simulink model "fig85_Lampara_CFL"  (R2021a)
settings: Solver=FixedStepAuto  StartTime=0.0  StopTime=tf  FixedStep=Ts  RelTol=1e-3  EnableMultiTasking=on
InitFcn:
  | %leer señal de archivos de Excel
  | %datos = textread('Lampara_CFL.txt');
  |  datos = [
  | -1.00E-02	-2.787500E+01	1.484375E-02
  | -9.95E-03	-3.271875E+01	2.531250E-02
  | -9.90E-03	-3.375000E+01	1.015625E-02
  | -9.85E-03	-3.593750E+01	1.562500E-04
  | -9.80E-03	-4.103125E+01	1.531250E-02
  | -9.75E-03	-4.600000E+01	1.015625E-02
  | -9.70E-03	-4.828125E+01	1.562500E-04
  | -9.65E-03	-4.850000E+01	2.031250E-02
  | -9.60E-03	-5.343750E+01	1.984375E-02
  | -9.55E-03	-5.646875E+01	9.687500E-03
  | -9.50E-03	-5.756250E+01	1.046875E-02
  | -9.45E-03	-6.150000E+01	1.046875E-02
  | -9.40E-03	-6.628125E+01	9.687500E-03
  | -9.35E-03	-6.834375E+01	-1.421875E-02
  | -9.30E-03	-6.840625E+01	-3.906250E-03
  | -9.25E-03	-7.328125E+01	2.468750E-02
  | -9.20E-03	-7.637500E+01	1.500000E-02
  | -9.15E-03	-7.443750E+01	1.484375E-02
  | -9.10E-03	-7.643750E+01	3.921875E-02
  | -9.05E-03	-8.156250E+01	3.453125E-02
  | -9.00E-03	-8.156250E+01	1.953125E-02
  | -8.95E-03	-8.356250E+01	3.453125E-02
  | -8.90E-03	-8.846875E+01	2.500000E-02
  | -8.85E-03	-9.050000E+01	7.812500E-04
  | -8.80E-03	-9.550000E+01	7.812500E-04
  | -8.75E-03	-9.837500E+01	1.015625E-02
  | -8.70E-03	-1.014688E+02	-9.062500E-03
  | -8.65E-03	-1.065000E+02	-1.906250E-02
  | -8.60E-03	-1.044688E+02	-9.687500E-03
  | -8.55E-03	-1.044688E+02	-3.937500E-02
  | -8.50E-03	-1.085625E+02	-8.453125E-02
  | -8.45E-03	-1.065625E+02	-1.485938E-01
  | -8.40E-03	-1.054375E+02	-2.331250E-01
  | -8.35E-03	-1.084063E+02	-3.331250E-01
  | -8.30E-03	-1.100313E+02	-4.517188E-01
  | -8.25E-03	-1.107188E+02	-5.465625E-01
  | -8.20E-03	-1.127188E+02	-6.164063E-01
  | -8.15E-03	-1.171875E+02	-6.709375E-01
  | -8.10E-03	-1.199375E+02	-6.857813E-01
  | -8.05E-03	-1.218750E+02	-6.804688E-01
  | -8.00E-03	-1.247813E+02	-6.517188E-01
  | -7.95E-03	-1.276875E+02	-5.914063E-01
  | -7.90E-03	-1.295000E+02	-5.362500E-01
  | -7.85E-03	-1.305625E+02	-4.728125E-01
  | -7.80E-03	-1.325625E+02	-4.084375E-01
  | -7.75E-03	-1.345313E+02	-3.642188E-01
  | -7.70E-03	-1.366875E+02	-3.250000E-01
  | -7.65E-03	-1.366875E+02	-3.145313E-01
  | -7.60E-03	-1.387500E+02	-3.187500E-01
  | -7.55E-03	-1.427813E+02	-3.195313E-01
  | -7.50E-03	-1.425938E+02	-3.439063E-01
  | -7.45E-03	-1.436563E+02	-3.578125E-01
  | -7.40E-03	-1.466563E+02	-3.631250E-01
  | -7.35E-03	-1.465938E+02	-3.785938E-01
  | -7.30E-03	-1.466563E+02	-3.785938E-01
  | -7.25E-03	-1.495938E+02	-3.734375E-01
  | -7.20E-03	-1.495625E+02	-3.682813E-01
  | -7.15E-03	-1.485000E+02	-3.487500E-01
  | -7.10E-03	-1.524375E+02	-3.343750E-01
  | -7.05E-03	-1.545000E+02	-3.240625E-01
  | -7.00E-03	-1.525625E+02	-2.943750E-01
  | -6.95E-03	-1.525938E+02	-2.706250E-01
  | -6.90E-03	-1.537500E+02	-2.660938E-01
  | -6.85E-03	-1.547813E+02	-2.456250E-01
  | -6.80E-03	-1.566563E+02	-2.204688E-01
  | -6.75E-03	-1.556250E+02	-2.057813E-01
  | -6.70E-03	-1.575313E+02	-1.850000E-01
  | -6.65E-03	-1.604375E+02	-1.596875E-01
  | -6.60E-03	-1.574063E+02	-1.393750E-01
  | -6.55E-03	-1.574063E+02	-1.246875E-01
  | -6.50E-03	-1.605000E+02	-9.562500E-02
  | -6.45E-03	-1.585000E+02	-6.046875E-02
  | -6.40E-03	-1.554063E+02	-3.593750E-02
  | -6.35E-03	-1.595313E+02	-2.171875E-02
  | -6.30E-03	-1.584688E+02	-6.093750E-03
  | -6.25E-03	-1.554063E+02	4.531250E-03
  | -6.20E-03	-1.574688E+02	4.531250E-03
  | -6.15E-03	-1.564375E+02	-1.562500E-04
  | -6.10E-03	-1.553750E+02	-4.843750E-03
  | -6.05E-03	-1.554063E+02	5.000000E-03
  | -6.00E-03	-1.564375E+02	1.437500E-02
  | -5.95E-03	-1.554063E+02	1.906250E-02
  | -5.90E-03	-1.533438E+02	3.921875E-02
  | -5.85E-03	-1.543438E+02	3.875000E-02
  | -5.80E-03	-1.553750E+02	3.375000E-02
  | -5.75E-03	-1.543438E+02	4.390625E-02
  | -5.70E-03	-1.533438E+02	2.875000E-02
  | -5.65E-03	-1.524063E+02	2.421875E-02
  | -5.60E-03	-1.505000E+02	2.953125E-02
  | -5.55E-03	-1.486563E+02	1.953125E-02
  | -5.50E-03	-1.466875E+02	1.484375E-02
  | -5.45E-03	-1.447813E+02	1.484375E-02
  | -5.40E-03	-1.458125E+02	5.468750E-03
  | -5.35E-03	-1.447500E+02	5.468750E-03
  | -5.30E-03	-1.428750E+02	9.687500E-03
  | -5.25E-03	-1.447813E+02	3.125000E-04
  | -5.20E-03	-1.426250E+02	1.062500E-02
  | -5.15E-03	-1.396875E+02	1.484375E-02
  | -5.10E-03	-1.385938E+02	1.484375E-02
  | -5.05E-03	-1.375313E+02	2.000000E-02
  | -5.00E-03	-1.355625E+02	9.687500E-03
  | -4.95E-03	-1.335625E+02	4.843750E-03
  | -4.90E-03	-1.344688E+02	1.500000E-02
  | -4.85E-03	-1.337188E+02	1.468750E-02
  | -4.80E-03	-1.329688E+02	-3.125000E-04
  | -4.75E-03	-1.357188E+02	9.843750E-03
  | -4.70E-03	-1.328438E+02	1.984375E-02
  | -4.65E-03	-1.301250E+02	9.687500E-03
  | -4.60E-03	-1.330000E+02	-3.125000E-04
  | -4.55E-03	-1.289375E+02	1.500000E-02
  | -4.50E-03	-1.250313E+02	1.984375E-02
  | -4.45E-03	-1.260625E+02	-5.468750E-03
  | -4.40E-03	-1.242188E+02	4.687500E-03
  | -4.35E-03	-1.223438E+02	1.953125E-02
  | -4.30E-03	-1.206563E+02	4.218750E-03
  | -4.25E-03	-1.190625E+02	4.218750E-03
  | -4.20E-03	-1.171875E+02	1.437500E-02
  | -4.15E-03	-1.155000E+02	4.218750E-03
  | -4.10E-03	-1.137500E+02	4.218750E-03
  | -4.05E-03	-1.086875E+02	9.375000E-03
  | -4.00E-03	-1.086875E+02	4.218750E-03
  | -3.95E-03	-1.077188E+02	-9.375000E-04
  | -3.90E-03	-1.037188E+02	4.218750E-03
  | -3.85E-03	-1.017500E+02	1.437500E-02
  | -3.80E-03	-9.671875E+01	4.218750E-03
  | -3.75E-03	-9.468750E+01	-9.375000E-04
  | -3.70E-03	-9.162500E+01	-9.375000E-04
  | -3.65E-03	-8.553125E+01	4.218750E-03
  | -3.60E-03	-8.350000E+01	-9.375000E-04
  | -3.55E-03	-8.143750E+01	-6.093750E-03
  | -3.50E-03	-7.840625E+01	1.875000E-02
  | -3.45E-03	-7.546875E+01	2.328125E-02
  | -3.40E-03	-7.353125E+01	1.375000E-02
  | -3.35E-03	-7.159375E+01	1.890625E-02
  | -3.30E-03	-6.759375E+01	1.828125E-02
  | -3.25E-03	-6.665625E+01	8.750000E-03
  | -3.20E-03	-6.378125E+01	9.375000E-03
  | -3.15E-03	-5.981250E+01	4.218750E-03
  | -3.10E-03	-5.981250E+01	-7.812500E-04
  | -3.05E-03	-5.371875E+01	1.437500E-02
  | -3.00E-03	-4.659375E+01	1.437500E-02
  | -2.95E-03	-4.753125E+01	4.531250E-03
  | -2.90E-03	-4.531250E+01	1.437500E-02
  | -2.85E-03	-3.809375E+01	9.375000E-03
  | -2.80E-03	-3.700000E+01	-4.687500E-04
  | -2.75E-03	-3.706250E+01	4.375000E-03
  | -2.70E-03	-3.221875E+01	-4.687500E-04
  | -2.65E-03	-2.925000E+01	-4.687500E-04
  | -2.60E-03	-2.931250E+01	-4.687500E-04
  | -2.55E-03	-2.746875E+01	4.375000E-03
  | -2.50E-03	-2.259375E+01	1.437500E-02
  | -2.45E-03	-2.153125E+01	1.437500E-02
  | -2.40E-03	-2.240625E+01	1.437500E-02
  | -2.35E-03	-1.550000E+01	1.937500E-02
  | -2.30E-03	-9.437500E+00	2.890625E-02
  | -2.25E-03	-7.437500E+00	1.390625E-02
  | -2.20E-03	-2.531250E+00	-4.687500E-04
  | -2.15E-03	1.437500E+00	9.062500E-03
  | -2.10E-03	5.156250E+00	4.062500E-03
  | -2.05E-03	7.875000E+00	-9.375000E-04
  | -2.00E-03	9.000000E+00	-5.781250E-03
  | -1.95E-03	1.181250E+01	-9.375000E-04
  | -1.90E-03	1.356250E+01	1.812500E-02
  | -1.85E-03	1.375000E+01	4.062500E-03
  | -1.80E-03	1.484375E+01	-5.000000E-03
  | -1.75E-03	1.678125E+01	4.531250E-03
  | -1.70E-03	1.878125E+01	-4.687500E-03
  | -1.65E-03	2.168750E+01	-1.421875E-02
  | -1.60E-03	2.456250E+01	-5.000000E-03
  | -1.55E-03	2.959375E+01	9.375000E-03
  | -1.50E-03	3.446875E+01	4.531250E-03
  | -1.45E-03	3.731250E+01	4.062500E-03
  | -1.40E-03	4.143750E+01	2.812500E-02
  | -1.35E-03	4.440625E+01	2.812500E-02
  | -1.30E-03	4.728125E+01	1.859375E-02
  | -1.25E-03	4.940625E+01	2.359375E-02
  | -1.20E-03	5.040625E+01	1.859375E-02
  | -1.15E-03	5.231250E+01	2.312500E-02
  | -1.10E-03	5.631250E+01	1.859375E-02
  | -1.05E-03	5.818750E+01	9.062500E-03
  | -1.00E-03	5.912500E+01	1.812500E-02
  | -9.50E-04	6.403125E+01	1.359375E-02
  | -9.00E-04	6.900000E+01	1.859375E-02
  | -8.50E-04	7.303125E+01	2.765625E-02
  | -8.00E-04	7.403125E+01	1.812500E-02
  | -7.50E-04	7.621875E+01	2.312500E-02
  | -7.00E-04	8.128125E+01	2.765625E-02
  | -6.50E-04	8.240625E+01	1.359375E-02
  | -6.00E-04	8.146875E+01	9.062500E-03
  | -5.50E-04	8.340625E+01	1.359375E-02
  | -5.00E-04	8.653125E+01	-1.562500E-04
  | -4.50E-04	8.746875E+01	3.125000E-04
  | -4.00E-04	9.037500E+01	4.843750E-03
  | -3.50E-04	9.334375E+01	-4.687500E-03
  | -3.00E-04	9.318750E+01	4.843750E-03
  | -2.50E-04	9.712500E+01	1.515625E-02
  | -2.00E-04	9.909375E+01	5.015625E-02
  | -1.50E-04	9.606250E+01	1.189063E-01
  | -1.00E-04	9.809375E+01	1.842188E-01
  | -5.00E-05	1.011875E+02	2.790625E-01
  | 0.00E+00	9.915625E+01	4.071875E-01
  | 5.00E-05	1.001563E+02	5.062500E-01
  | 1.00E-04	1.062813E+02	5.756250E-01
  | 1.50E-04	1.074688E+02	6.493750E-01
  | 2.00E-04	1.077500E+02	6.881250E-01
  | 2.50E-04	1.136563E+02	6.929688E-01
  | 3.00E-04	1.177500E+02	6.739063E-01
  | 3.50E-04	1.199063E+02	6.246875E-01
  | 4.00E-04	1.236563E+02	5.898438E-01
  | 4.50E-04	1.267500E+02	5.160938E-01
  | 5.00E-04	1.286250E+02	4.479688E-01
  | 5.50E-04	1.296875E+02	3.882813E-01
  | 6.00E-04	1.300938E+02	3.834375E-01
  | 6.50E-04	1.300938E+02	3.590625E-01
  | 7.00E-04	1.304688E+02	3.440625E-01
  | 7.50E-04	1.304688E+02	3.489063E-01
  | 8.00E-04	1.323750E+02	3.342188E-01
  | 8.50E-04	1.346563E+02	3.587500E-01
  | 9.00E-04	1.354688E+02	3.637500E-01
  | 9.50E-04	1.374375E+02	3.840625E-01
  | 1.00E-03	1.397188E+02	3.890625E-01
  | 1.05E-03	1.407813E+02	3.840625E-01
  | 1.10E-03	1.408750E+02	3.742188E-01
  | 1.15E-03	1.448750E+02	3.581250E-01
  | 1.20E-03	1.488125E+02	3.479688E-01
  | 1.25E-03	1.478750E+02	3.431250E-01
  | 1.30E-03	1.498438E+02	3.065625E-01
  | 1.35E-03	1.535938E+02	2.915625E-01
  | 1.40E-03	1.535938E+02	2.868750E-01
  | 1.45E-03	1.509063E+02	2.617188E-01
  | 1.50E-03	1.518125E+02	2.470313E-01
  | 1.55E-03	1.545625E+02	2.281250E-01
  | 1.60E-03	1.517500E+02	2.143750E-01
  | 1.65E-03	1.507188E+02	2.092188E-01
  | 1.70E-03	1.516250E+02	1.845313E-01
  | 1.75E-03	1.496875E+02	1.553125E-01
  | 1.80E-03	1.486563E+02	1.304688E-01
  | 1.85E-03	1.496875E+02	1.053125E-01
  | 1.90E-03	1.496875E+02	7.484375E-02
  | 1.95E-03	1.496563E+02	3.984375E-02
  | 2.00E-03	1.517188E+02	2.000000E-02
  | 2.05E-03	1.536563E+02	1.500000E-02
  | 2.10E-03	1.566875E+02	9.843750E-03
  | 2.15E-03	1.568750E+02	-1.078125E-02
  | 2.20E-03	1.547813E+02	-1.578125E-02
  | 2.25E-03	1.556875E+02	-4.687500E-04
  | 2.30E-03	1.557813E+02	-5.781250E-03
  | 2.35E-03	1.517188E+02	-2.140625E-02
  | 2.40E-03	1.477813E+02	-2.140625E-02
  | 2.45E-03	1.486875E+02	-5.781250E-03
  | 2.50E-03	1.467188E+02	-1.109375E-02
  | 2.55E-03	1.448438E+02	-2.671875E-02
  | 2.60E-03	1.446563E+02	-1.640625E-02
  | 2.65E-03	1.416250E+02	-1.640625E-02
  | 2.70E-03	1.426250E+02	-1.640625E-02
  | 2.75E-03	1.406875E+02	-1.140625E-02
  | 2.80E-03	1.407188E+02	-1.140625E-02
  | 2.85E-03	1.428438E+02	-7.812500E-04
  | 2.90E-03	1.411250E+02	-1.109375E-02
  | 2.95E-03	1.440000E+02	-1.640625E-02
  | 3.00E-03	1.420313E+02	-6.093750E-03
  | 3.05E-03	1.392188E+02	-1.109375E-02
  | 3.10E-03	1.410000E+02	-1.109375E-02
  | 3.15E-03	1.369375E+02	-1.140625E-02
  | 3.20E-03	1.340938E+02	-7.812500E-04
  | 3.25E-03	1.360313E+02	9.843750E-03
  | 3.30E-03	1.358750E+02	4.531250E-03
  | 3.35E-03	1.330313E+02	-3.125000E-04
  | 3.40E-03	1.331875E+02	-5.781250E-03
  | 3.45E-03	1.329688E+02	1.000000E-02
  | 3.50E-03	1.299375E+02	5.000000E-03
  | 3.55E-03	1.290313E+02	4.218750E-03
  | 3.60E-03	1.299375E+02	2.531250E-02
  | 3.65E-03	1.288438E+02	2.546875E-02
  | 3.70E-03	1.256563E+02	3.000000E-02
  | 3.75E-03	1.253750E+02	3.062500E-02
  | 3.80E-03	1.253750E+02	2.546875E-02
  | 3.85E-03	1.232813E+02	2.015625E-02
  | 3.90E-03	1.199375E+02	2.078125E-02
  | 3.95E-03	1.177500E+02	2.078125E-02
  | 4.00E-03	1.158125E+02	2.078125E-02
  | 4.05E-03	1.138125E+02	2.078125E-02
  | 4.10E-03	1.105625E+02	2.078125E-02
  | 4.15E-03	1.045625E+02	1.531250E-02
  | 4.20E-03	1.046875E+02	4.375000E-03
  | 4.25E-03	1.036250E+02	1.468750E-02
  | 4.30E-03	9.862500E+01	-1.406250E-03
  | 4.35E-03	9.762500E+01	-1.171875E-02
  | 4.40E-03	9.559375E+01	9.218750E-03
  | 4.45E-03	9.465625E+01	-1.406250E-03
  | 4.50E-03	9.156250E+01	-9.375000E-04
  | 4.55E-03	8.643750E+01	9.843750E-03
  | 4.60E-03	8.656250E+01	1.937500E-02
  | 4.65E-03	8.462500E+01	2.484375E-02
  | 4.70E-03	7.862500E+01	4.375000E-03
  | 4.75E-03	7.568750E+01	-1.718750E-03
  | 4.80E-03	7.375000E+01	-1.718750E-03
  | 4.85E-03	7.084375E+01	-6.406250E-03
  | 4.90E-03	6.887500E+01	-1.187500E-02
  | 4.95E-03	6.596875E+01	-1.187500E-02
  | 5.00E-03	6.409375E+01	-9.375000E-04
  | 5.05E-03	6.315625E+01	1.406250E-02
  | 5.10E-03	5.906250E+01	8.593750E-03
  | 5.15E-03	5.593750E+01	-9.375000E-04
  | 5.20E-03	5.493750E+01	9.218750E-03
  | 5.25E-03	5.175000E+01	-1.562500E-03
  | 5.30E-03	4.956250E+01	3.437500E-03
  | 5.35E-03	4.671875E+01	1.437500E-02
  | 5.40E-03	4.481250E+01	3.750000E-03
  | 5.45E-03	4.284375E+01	1.859375E-02
  | 5.50E-03	3.806250E+01	2.390625E-02
  | 5.55E-03	3.525000E+01	9.218750E-03
  | 5.60E-03	3.231250E+01	9.218750E-03
  | 5.65E-03	2.828125E+01	1.406250E-02
  | 5.70E-03	2.434375E+01	4.531250E-03
  | 5.75E-03	2.137500E+01	-5.156250E-03
  | 5.80E-03	1.831250E+01	-3.125000E-04
  | 5.85E-03	1.534375E+01	9.531250E-03
  | 5.90E-03	1.334375E+01	-1.562500E-04
  | 5.95E-03	1.034375E+01	-1.000000E-02
  | 6.00E-03	6.437500E+00	9.843750E-03
  | 6.05E-03	3.593750E+00	9.843750E-03
  | 6.10E-03	7.187500E-01	0.000000E+00
  | 6.15E-03	-2.218750E+00	5.000000E-03
  | 6.20E-03	-5.250000E+00	4.687500E-03
  | 6.25E-03	-7.250000E+00	9.531250E-03
  | 6.30E-03	-9.062500E+00	4.687500E-03
  | 6.35E-03	-1.296875E+01	4.687500E-03
  | 6.40E-03	-1.600000E+01	9.531250E-03
  | 6.45E-03	-1.781250E+01	9.531250E-03
  | 6.50E-03	-2.368750E+01	9.843750E-03
  | 6.55E-03	-2.753125E+01	-3.125000E-04
  | 6.60E-03	-2.753125E+01	-6.250000E-04
  | 6.65E-03	-3.359375E+01	-5.468750E-03
  | 6.70E-03	-3.743750E+01	-2.046875E-02
  | 6.75E-03	-3.553125E+01	-1.046875E-02
  | 6.80E-03	-3.853125E+01	4.531250E-03
  | 6.85E-03	-4.540625E+01	-1.046875E-02
  | 6.90E-03	-4.643750E+01	-1.531250E-02
  | 6.95E-03	-4.546875E+01	4.687500E-03
  | 7.00E-03	-5.134375E+01	-6.250000E-04
  | 7.05E-03	-5.712500E+01	-1.046875E-02
  | 7.10E-03	-5.721875E+01	-3.125000E-04
  | 7.15E-03	-5.918750E+01	-6.250000E-04
  | 7.20E-03	-6.300000E+01	-5.468750E-03
  | 7.25E-03	-6.600000E+01	4.687500E-03
  | 7.30E-03	-6.800000E+01	4.531250E-03
  | 7.35E-03	-7.015625E+01	-1.046875E-02
  | 7.40E-03	-7.537500E+01	-3.125000E-04
  | 7.45E-03	-7.515625E+01	-6.250000E-04
  | 7.50E-03	-7.421875E+01	-1.078125E-02
  | 7.55E-03	-8.165625E+01	-5.625000E-03
  | 7.60E-03	-8.450000E+01	-5.625000E-03
  | 7.65E-03	-8.240625E+01	-6.250000E-04
  | 7.70E-03	-8.659375E+01	4.531250E-03
  | 7.75E-03	-9.156250E+01	-6.250000E-04
  | 7.80E-03	-9.362500E+01	-6.250000E-04
  | 7.85E-03	-9.565625E+01	4.531250E-03
  | 7.90E-03	-9.756250E+01	-6.250000E-04
  | 7.95E-03	-9.959375E+01	-5.625000E-03
  | 8.00E-03	-1.006563E+02	-5.625000E-03
  | 8.05E-03	-1.025313E+02	-5.625000E-03
  | 8.10E-03	-1.044375E+02	-2.125000E-02
  | 8.15E-03	-1.035000E+02	-6.125000E-02
  | 8.20E-03	-1.043750E+02	-1.154688E-01
  | 8.25E-03	-1.072500E+02	-1.965625E-01
  | 8.30E-03	-1.083125E+02	-3.007813E-01
  | 8.35E-03	-1.082813E+02	-4.087500E-01
  | 8.40E-03	-1.104375E+02	-5.192188E-01
  | 8.45E-03	-1.136250E+02	-5.989063E-01
  | 8.50E-03	-1.136563E+02	-6.526563E-01
  | 8.55E-03	-1.167188E+02	-6.971875E-01
  | 8.60E-03	-1.189063E+02	-6.973438E-01
  | 8.65E-03	-1.199688E+02	-6.631250E-01
  | 8.70E-03	-1.246875E+02	-6.184375E-01
  | 8.75E-03	-1.276563E+02	-5.640625E-01
  | 8.80E-03	-1.316875E+02	-4.990625E-01
  | 8.85E-03	-1.325938E+02	-4.392188E-01
  | 8.90E-03	-1.345938E+02	-3.953125E-01
  | 8.95E-03	-1.395313E+02	-3.546875E-01
  | 9.00E-03	-1.385313E+02	-3.289063E-01
  | 9.05E-03	-1.375313E+02	-3.242188E-01
  | 9.10E-03	-1.415313E+02	-3.192188E-01
  | 9.15E-03	-1.435625E+02	-3.343750E-01
  | 9.20E-03	-1.405938E+02	-3.492188E-01
  | 9.25E-03	-1.425938E+02	-3.548438E-01
  | 9.30E-03	-1.466250E+02	-3.862500E-01
  | 9.35E-03	-1.445938E+02	-3.959375E-01
  | 9.40E-03	-1.453438E+02	-4.014063E-01
  | 9.45E-03	-1.483438E+02	-3.967188E-01
  | 9.50E-03	-1.492813E+02	-3.607813E-01
  | 9.55E-03	-1.508125E+02	-3.414063E-01
  | 9.60E-03	-1.516250E+02	-3.256250E-01
  | 9.65E-03	-1.508438E+02	-2.895313E-01
  | 9.70E-03	-1.516250E+02	-2.507813E-01
  | 9.75E-03	-1.540000E+02	-2.559375E-01
  | 9.80E-03	-1.542813E+02	-2.506250E-01
  | 9.85E-03	-1.553125E+02	-2.157813E-01
  | 9.90E-03	-1.558750E+02	-2.062500E-01
  | 9.95E-03	-1.569063E+02	-1.960938E-01
  | 1.00E-02	-1.600313E+02	-1.664063E-01
  | 1.01E-02	-1.579688E+02	-1.421875E-01
  | 1.01E-02	-1.569063E+02	-1.371875E-01
  | 1.02E-02	-1.610938E+02	-1.070313E-01
  | 1.02E-02	-1.590313E+02	-7.203125E-02
  | 1.03E-02	-1.569063E+02	-7.203125E-02
  | 1.03E-02	-1.590000E+02	-5.125000E-02
  | 1.04E-02	-1.569375E+02	-1.562500E-02
  | 1.04E-02	-1.550625E+02	-1.078125E-02
  | 1.05E-02	-1.550625E+02	-9.375000E-04
  | 1.05E-02	-1.558750E+02	9.218750E-03
  | 1.06E-02	-1.552188E+02	1.406250E-02
  | 1.06E-02	-1.551563E+02	1.875000E-02
  | 1.07E-02	-1.588750E+02	4.531250E-03
  | 1.07E-02	-1.590313E+02	9.375000E-03
  | 1.08E-02	-1.554063E+02	2.375000E-02
  | 1.08E-02	-1.564375E+02	1.406250E-02
  | 1.09E-02	-1.573750E+02	4.375000E-03
  | 1.09E-02	-1.530625E+02	2.375000E-02
  | 1.10E-02	-1.502500E+02	2.828125E-02
  | 1.10E-02	-1.502500E+02	4.375000E-03
  | 1.11E-02	-1.514688E+02	9.375000E-03
  | 1.11E-02	-1.494688E+02	9.375000E-03
  | 1.12E-02	-1.465313E+02	-4.843750E-03
  | 1.12E-02	-1.485313E+02	-1.562500E-04
  | 1.13E-02	-1.495938E+02	9.375000E-03
  | 1.13E-02	-1.455625E+02	9.375000E-03
  | 1.14E-02	-1.434375E+02	9.062500E-03
  | 1.14E-02	-1.484375E+02	2.328125E-02
  | 1.15E-02	-1.474063E+02	2.328125E-02
  | 1.15E-02	-1.423125E+02	1.375000E-02
  | 1.16E-02	-1.442813E+02	1.375000E-02
  | 1.16E-02	-1.443438E+02	1.828125E-02
  | 1.17E-02	-1.393750E+02	2.328125E-02
  | 1.17E-02	-1.344375E+02	2.375000E-02
  | 1.18E-02	-1.353438E+02	1.406250E-02
  | 1.18E-02	-1.352188E+02	9.531250E-03
  | 1.19E-02	-1.322188E+02	1.453125E-02
  | 1.19E-02	-1.322500E+02	3.125000E-04
  | 1.20E-02	-1.331875E+02	-4.687500E-03
  | 1.20E-02	-1.331875E+02	-1.562500E-04
  | 1.21E-02	-1.304688E+02	-4.687500E-03
  | 1.21E-02	-1.273750E+02	9.062500E-03
  | 1.22E-02	-1.241875E+02	2.328125E-02
  | 1.22E-02	-1.232500E+02	1.875000E-02
  | 1.23E-02	-1.210625E+02	1.375000E-02
  | 1.23E-02	-1.168750E+02	2.328125E-02
  | 1.24E-02	-1.159375E+02	2.828125E-02
  | 1.24E-02	-1.140938E+02	9.531250E-03
  | 1.25E-02	-1.130625E+02	-4.843750E-03
  | 1.25E-02	-1.121563E+02	1.562500E-04
  | 1.26E-02	-1.082813E+02	3.125000E-04
  | 1.26E-02	-1.071875E+02	-1.875000E-02
  | 1.27E-02	-1.062188E+02	-1.375000E-02
  | 1.27E-02	-1.032500E+02	4.843750E-03
  | 1.28E-02	-9.912500E+01	1.562500E-04
  | 1.28E-02	-9.721875E+01	1.031250E-02
  | 1.29E-02	-9.625000E+01	1.953125E-02
  | 1.29E-02	-9.112500E+01	1.453125E-02
  | 1.30E-02	-8.903125E+01	1.953125E-02
  | 1.30E-02	-8.787500E+01	2.468750E-02
  | 1.31E-02	-8.384375E+01	1.453125E-02
  | 1.31E-02	-7.875000E+01	1.453125E-02
  | 1.32E-02	-7.759375E+01	3.000000E-02
  | 1.32E-02	-7.762500E+01	1.046875E-02
  | 1.33E-02	-7.078125E+01	1.562500E-04
  | 1.33E-02	-6.881250E+01	2.484375E-02
  | 1.34E-02	-6.981250E+01	2.093750E-02
  | 1.34E-02	-6.396875E+01	1.593750E-02
  | 1.35E-02	-6.093750E+01	1.515625E-02
  | 1.35E-02	-5.996875E+01	1.531250E-02
  | 1.36E-02	-5.600000E+01	3.546875E-02
  | 1.36E-02	-5.303125E+01	2.562500E-02
  | 1.37E-02	-5.212500E+01	4.843750E-03
  | 1.37E-02	-5.109375E+01	1.984375E-02
  | 1.38E-02	-4.812500E+01	3.000000E-02
  | 1.38E-02	-4.521875E+01	1.953125E-02
  | 1.39E-02	-4.328125E+01	1.953125E-02
  | 1.39E-02	-4.053125E+01	2.468750E-02
  | 1.40E-02	-3.671875E+01	2.468750E-02
  | 1.40E-02	-3.178125E+01	3.000000E-02
  | 1.41E-02	-3.006250E+01	4.468750E-02
  | 1.41E-02	-2.915625E+01	3.937500E-02
  | 1.42E-02	-2.612500E+01	2.484375E-02
  | 1.42E-02	-2.421875E+01	2.953125E-02
  | 1.43E-02	-2.112500E+01	2.421875E-02
  | 1.43E-02	-1.918750E+01	1.484375E-02
  | 1.44E-02	-1.728125E+01	-3.125000E-04
  | 1.44E-02	-1.128125E+01	-3.125000E-04
  | 1.45E-02	-5.312500E+00	1.515625E-02
  | 1.45E-02	-4.281250E+00	1.484375E-02
  | 1.46E-02	-1.312500E+00	9.687500E-03
  | 1.46E-02	4.625000E+00	4.687500E-03
  | 1.47E-02	8.625000E+00	2.937500E-02
  | 1.47E-02	1.056250E+01	2.953125E-02
  | 1.48E-02	1.343750E+01	1.000000E-02
  | 1.48E-02	1.840625E+01	1.953125E-02
  | 1.49E-02	1.937500E+01	1.453125E-02
  | 1.49E-02	2.125000E+01	1.531250E-02
  | 1.50E-02	2.521875E+01	1.000000E-02
  | 1.50E-02	2.734375E+01	-3.125000E-04
  | 1.51E-02	2.825000E+01	5.000000E-03
  | 1.51E-02	2.912500E+01	-3.125000E-04
  | 1.52E-02	3.431250E+01	-3.125000E-04
  | 1.52E-02	3.837500E+01	9.687500E-03
  | 1.53E-02	3.831250E+01	4.531250E-03
  | 1.53E-02	4.137500E+01	-1.062500E-02
  | 1.54E-02	4.834375E+01	4.375000E-03
  | 1.54E-02	5.037500E+01	1.984375E-02
  | 1.55E-02	4.946875E+01	1.484375E-02
  | 1.55E-02	5.518750E+01	9.531250E-03
  | 1.56E-02	5.918750E+01	2.953125E-02
  | 1.56E-02	5.825000E+01	3.953125E-02
  | 1.57E-02	6.106250E+01	9.531250E-03
  | 1.57E-02	6.703125E+01	2.437500E-02
  | 1.58E-02	6.796875E+01	3.484375E-02
  | 1.58E-02	6.796875E+01	1.484375E-02
  | 1.59E-02	7.190625E+01	2.953125E-02
  | 1.59E-02	7.490625E+01	4.000000E-02
  | 1.60E-02	7.696875E+01	2.468750E-02
  | 1.60E-02	7.790625E+01	1.875000E-02
  | 1.61E-02	8.087500E+01	1.875000E-02
  | 1.61E-02	8.293750E+01	3.906250E-03
  | 1.62E-02	8.400000E+01	-1.406250E-03
  | 1.62E-02	8.921875E+01	-6.718750E-03
  | 1.63E-02	9.040625E+01	-6.093750E-03
  | 1.63E-02	9.037500E+01	-1.093750E-03
  | 1.64E-02	9.668750E+01	-6.406250E-03
  | 1.64E-02	9.787500E+01	8.593750E-03
  | 1.65E-02	9.478125E+01	2.781250E-02
  | 1.65E-02	9.787500E+01	7.281250E-02
  | 1.66E-02	9.800000E+01	1.526563E-01
  | 1.66E-02	9.590625E+01	2.501563E-01
  | 1.67E-02	9.896875E+01	3.692188E-01
  | 1.67E-02	1.001563E+02	4.693750E-01
  | 1.68E-02	1.011250E+02	5.671875E-01
  | 1.68E-02	1.050313E+02	6.560938E-01
  | 1.69E-02	1.069688E+02	6.914063E-01
  | 1.69E-02	1.100000E+02	6.859375E-01
  | 1.70E-02	1.138750E+02	6.709375E-01
  | 1.70E-02	1.158750E+02	6.364063E-01
  | 1.71E-02	1.199375E+02	5.714063E-01
  | 1.71E-02	1.207813E+02	5.175000E-01
  | 1.72E-02	1.209063E+02	4.687500E-01
  | 1.72E-02	1.250938E+02	4.237500E-01
  | 1.73E-02	1.268125E+02	3.800000E-01
  | 1.73E-02	1.267188E+02	3.462500E-01
  | 1.74E-02	1.288125E+02	3.414063E-01
  | 1.74E-02	1.335625E+02	3.414063E-01
  | 1.75E-02	1.344688E+02	3.362500E-01
  | 1.75E-02	1.354688E+02	3.364063E-01
  | 1.76E-02	1.364375E+02	3.709375E-01
  | 1.76E-02	1.373438E+02	3.804688E-01
  | 1.77E-02	1.412813E+02	3.707813E-01
  | 1.77E-02	1.374375E+02	3.904688E-01
  | 1.78E-02	1.383438E+02	3.856250E-01
  | 1.78E-02	1.422500E+02	3.709375E-01
  | 1.79E-02	1.411875E+02	3.660938E-01
  | 1.79E-02	1.431250E+02	3.612500E-01
  | 1.80E-02	1.431563E+02	3.360938E-01
  | 1.80E-02	1.440938E+02	3.060938E-01
  | 1.81E-02	1.450938E+02	3.012500E-01
  | 1.81E-02	1.462188E+02	2.860938E-01
  | 1.82E-02	1.482500E+02	2.567188E-01
  | 1.82E-02	1.482500E+02	2.375000E-01
  | 1.83E-02	1.502813E+02	2.323438E-01
  | 1.83E-02	1.532500E+02	2.281250E-01
  | 1.84E-02	1.552500E+02	2.037500E-01
  | 1.84E-02	1.552500E+02	1.784375E-01
  | 1.85E-02	1.541875E+02	1.678125E-01
  | 1.85E-02	1.541563E+02	1.279688E-01
  | 1.86E-02	1.541563E+02	8.828125E-02
  | 1.86E-02	1.541875E+02	6.781250E-02
  | 1.87E-02	1.519688E+02	2.859375E-02
  | 1.87E-02	1.508438E+02	4.375000E-03
  | 1.88E-02	1.541563E+02	-9.375000E-04
  | 1.88E-02	1.530313E+02	-7.812500E-04
  | 1.89E-02	1.488125E+02	4.531250E-03
  | 1.89E-02	1.510000E+02	3.906250E-03
  | 1.90E-02	1.519688E+02	2.312500E-02
  | 1.90E-02	1.509375E+02	2.843750E-02
  | 1.91E-02	1.509375E+02	2.343750E-02
  | 1.91E-02	1.507813E+02	3.781250E-02
  | 1.92E-02	1.499688E+02	2.828125E-02
  | 1.92E-02	1.480625E+02	1.859375E-02
  | 1.93E-02	1.479688E+02	2.343750E-02
  | 1.93E-02	1.431250E+02	8.593750E-03
  | 1.94E-02	1.430625E+02	-1.125000E-02
  | 1.94E-02	1.460313E+02	-1.250000E-03
  | 1.95E-02	1.402500E+02	-6.250000E-03
  | 1.95E-02	1.411875E+02	-2.125000E-02
  | 1.96E-02	1.450625E+02	-5.937500E-03
  | 1.96E-02	1.411875E+02	3.906250E-03
  | 1.97E-02	1.393438E+02	1.343750E-02
  | 1.97E-02	1.403125E+02	1.390625E-02
  | 1.98E-02	1.392813E+02	9.218750E-03
  | 1.98E-02	1.373750E+02	8.593750E-03
  | 1.99E-02	1.364063E+02	-6.250000E-03
  | 1.99E-02	1.325938E+02	-1.031250E-02
  | 2.00E-02	1.316563E+02	-1.031250E-02
  | 2.00E-02	1.335938E+02	-6.250000E-03
  | 2.01E-02	1.288750E+02	3.906250E-03
  | 2.01E-02	1.289063E+02	-7.812500E-04
  | 2.02E-02	1.308750E+02	8.593750E-03
  | 2.02E-02	1.269063E+02	1.875000E-02
  | 2.03E-02	1.257813E+02	-1.406250E-03
  | 2.03E-02	1.247500E+02	-1.140625E-02
  | 2.04E-02	1.206875E+02	-6.093750E-03
  | 2.04E-02	1.195938E+02	-1.656250E-02
  | 2.05E-02	1.194688E+02	-1.656250E-02
  | 2.05E-02	1.165938E+02	-6.093750E-03
  | 2.06E-02	1.147813E+02	-1.125000E-02
  | 2.06E-02	1.148438E+02	4.218750E-03
  | 2.07E-02	1.128438E+02	1.984375E-02
  | 2.07E-02	1.089375E+02	9.843750E-03
  | 2.08E-02	1.080625E+02	1.453125E-02
  | 2.08E-02	1.070000E+02	1.984375E-02
  | 2.09E-02	1.038125E+02	-6.250000E-04
  | 2.09E-02	1.038125E+02	-1.125000E-02
  | 2.10E-02	1.006250E+02	-6.093750E-03
  | 2.10E-02	9.868750E+01	-1.125000E-02
  | 2.11E-02	9.762500E+01	-1.656250E-02
  | 2.11E-02	9.106250E+01	-1.671875E-02
  | 2.12E-02	8.921875E+01	-7.812500E-04
  | 2.12E-02	8.721875E+01	9.843750E-03
  | 2.13E-02	8.290625E+01	-7.812500E-04
  | 2.13E-02	7.993750E+01	4.531250E-03
  | 2.14E-02	7.800000E+01	1.000000E-02
  | 2.14E-02	7.618750E+01	4.687500E-03
  | 2.15E-02	7.209375E+01	4.531250E-03
  | 2.15E-02	7.003125E+01	-6.250000E-04
  | 2.16E-02	6.612500E+01	-6.250000E-04
  | 2.16E-02	6.200000E+01	4.531250E-03
  | 2.17E-02	6.190625E+01	-6.250000E-04
  | 2.17E-02	5.787500E+01	-5.625000E-03
  | 2.18E-02	5.496875E+01	4.687500E-03
  | 2.18E-02	5.700000E+01	1.000000E-02
  | 2.19E-02	5.693750E+01	-3.125000E-04
  | 2.19E-02	5.421875E+01	-3.125000E-04
  | 2.20E-02	5.137500E+01	5.000000E-03
  | 2.20E-02	4.931250E+01	1.000000E-02
  | 2.21E-02	4.543750E+01	-5.000000E-03
  | 2.21E-02	4.046875E+01	-1.000000E-02
  | 2.22E-02	3.746875E+01	1.531250E-02
  | 2.22E-02	3.334375E+01	3.125000E-04
  | 2.23E-02	3.225000E+01	-1.000000E-02
  | 2.23E-02	3.040625E+01	4.687500E-04
  | 2.24E-02	2.634375E+01	5.468750E-03
  | 2.24E-02	2.634375E+01	1.562500E-04
  | 2.25E-02	2.250000E+01	-4.531250E-03
  | 2.25E-02	1.956250E+01	1.546875E-02
  | 2.26E-02	1.562500E+01	1.515625E-02
  | 2.26E-02	9.625000E+00	1.515625E-02
  | 2.27E-02	9.625000E+00	1.984375E-02
  | 2.27E-02	7.718750E+00	1.453125E-02
  | 2.28E-02	-3.125000E-01	9.531250E-03
  | 2.28E-02	-3.375000E+00	4.375000E-03
  | 2.29E-02	-3.281250E+00	-6.250000E-04
  | 2.29E-02	-8.281250E+00	-6.250000E-04
  | 2.30E-02	-1.231250E+01	-5.625000E-03
  | 2.30E-02	-1.715625E+01	-1.562500E-02
  | 2.31E-02	-2.003125E+01	-1.062500E-02
  | 2.31E-02	-2.112500E+01	-2.000000E-02
  | 2.32E-02	-2.206250E+01	-1.484375E-02
  | 2.32E-02	-2.290625E+01	-5.156250E-03
  | 2.33E-02	-2.706250E+01	-2.406250E-02
  | 2.33E-02	-2.881250E+01	9.375000E-04
  | 2.34E-02	-3.046875E+01	1.515625E-02
  | 2.34E-02	-3.456250E+01	-4.687500E-03
  | 2.35E-02	-4.128125E+01	1.015625E-02
  | 2.35E-02	-4.500000E+01	1.484375E-02
  | 2.36E-02	-4.415625E+01	4.531250E-03
  | 2.36E-02	-4.803125E+01	9.531250E-03
  | 2.37E-02	-5.096875E+01	4.843750E-03
  | 2.37E-02	-5.006250E+01	-4.687500E-03
  | 2.38E-02	-5.306250E+01	4.843750E-03
  | 2.38E-02	-5.884375E+01	1.515625E-02
  | 2.39E-02	-6.178125E+01	1.593750E-02
  | 2.39E-02	-6.293750E+01	5.625000E-03
  | 2.40E-02	-6.878125E+01	9.375000E-04
  | 2.40E-02	-7.365625E+01	1.593750E-02
  | 2.41E-02	-7.271875E+01	1.015625E-02
  | 2.41E-02	-7.468750E+01	-4.375000E-03
  | 2.42E-02	-7.962500E+01	-9.062500E-03
  | 2.42E-02	-8.056250E+01	-4.843750E-03
  | 2.43E-02	-8.056250E+01	4.843750E-03
  | 2.43E-02	-8.368750E+01	-4.375000E-03
  | 2.44E-02	-8.787500E+01	1.562500E-04
  | 2.44E-02	-8.900000E+01	4.843750E-03
  | 2.45E-02	-9.015625E+01	-1.562500E-04
  | 2.45E-02	-9.531250E+01	1.453125E-02
  | 2.46E-02	-9.834375E+01	2.953125E-02
  | 2.46E-02	-9.931250E+01	1.937500E-02
  | 2.47E-02	-1.002500E+02	4.843750E-03
  | 2.47E-02	-1.032500E+02	1.000000E-02
  | 2.48E-02	-1.053125E+02	-1.562500E-04
  | 2.48E-02	-1.043438E+02	-4.984375E-02
  | 2.49E-02	-1.054063E+02	-1.046875E-01
  | 2.49E-02	-1.055938E+02	-1.745313E-01
  | 2.50E-02	-1.055625E+02	-2.843750E-01
  | 2.50E-02	-1.065000E+02	-3.837500E-01
  | 2.51E-02	-1.074375E+02	-4.878125E-01
  | 2.51E-02	-1.093750E+02	-5.923438E-01
  | 2.52E-02	-1.113125E+02	-6.567188E-01
  | 2.52E-02	-1.142500E+02	-6.810938E-01
  | 2.53E-02	-1.192813E+02	-6.810938E-01
  | 2.53E-02	-1.214063E+02	-6.660938E-01
  | 2.54E-02	-1.225000E+02	-6.167188E-01
  | 2.54E-02	-1.283750E+02	-5.525000E-01
  | 2.55E-02	-1.323750E+02	-4.975000E-01
  | 2.55E-02	-1.335000E+02	-4.631250E-01
  | 2.56E-02	-1.342500E+02	-4.135938E-01
  | 2.56E-02	-1.361875E+02	-3.585938E-01
  | 2.57E-02	-1.383438E+02	-3.585938E-01
  | 2.57E-02	-1.393750E+02	-3.529688E-01
  | 2.58E-02	-1.404063E+02	-3.381250E-01
  | 2.58E-02	-1.394375E+02	-3.482813E-01
  | 2.59E-02	-1.425000E+02	-3.529688E-01
  | 2.59E-02	-1.465313E+02	-3.678125E-01
  | 2.60E-02	-1.455313E+02	-3.489063E-01
  | 2.60E-02	-1.445000E+02	-3.248438E-01
  | 2.61E-02	-1.454688E+02	-3.184375E-01
  | 2.61E-02	-1.492813E+02	-3.489063E-01
  | 2.62E-02	-1.528750E+02	-3.196875E-01
  | 2.62E-02	-1.526250E+02	-3.295313E-01
  | 2.63E-02	-1.535313E+02	-3.390625E-01
  | 2.63E-02	-1.573438E+02	-3.237500E-01
  | 2.64E-02	-1.580000E+02	-2.903125E-01
  | 2.64E-02	-1.559688E+02	-2.757813E-01
  | 2.65E-02	-1.561875E+02	-2.501563E-01
  | 2.65E-02	-1.570625E+02	-2.160938E-01
  | 2.66E-02	-1.568438E+02	-2.067188E-01
  | 2.66E-02	-1.578125E+02	-1.965625E-01
  | 2.67E-02	-1.609688E+02	-1.714063E-01
  | 2.67E-02	-1.630000E+02	-1.520313E-01
  | 2.68E-02	-1.598438E+02	-1.373438E-01
  | 2.68E-02	-1.610000E+02	-1.218750E-01
  | 2.69E-02	-1.641250E+02	-9.187500E-02
  | 2.69E-02	-1.599688E+02	-5.671875E-02
  | 2.70E-02	-1.590000E+02	-4.140625E-02
  | 2.70E-02	-1.590000E+02	-1.625000E-02
  | 2.71E-02	-1.590000E+02	3.750000E-03
  | 2.71E-02	-1.600313E+02	4.062500E-03
  | 2.72E-02	-1.569063E+02	1.843750E-02
  | 2.72E-02	-1.590313E+02	2.781250E-02
  | 2.73E-02	-1.600625E+02	8.750000E-03
  | 2.73E-02	-1.550625E+02	-6.250000E-03
  | 2.74E-02	-1.571563E+02	8.593750E-03
  | 2.74E-02	-1.590000E+02	9.218750E-03
  | 2.75E-02	-1.560938E+02	-5.781250E-03
  | 2.75E-02	-1.552813E+02	4.375000E-03
  | 2.76E-02	-1.543125E+02	9.531250E-03
  | 2.76E-02	-1.533438E+02	1.937500E-02
  | 2.77E-02	-1.515000E+02	1.937500E-02
  | 2.77E-02	-1.486563E+02	4.531250E-03
  | 2.78E-02	-1.486563E+02	9.531250E-03
  | 2.78E-02	-1.479375E+02	1.468750E-02
  | 2.79E-02	-1.479375E+02	2.437500E-02
  | 2.79E-02	-1.505938E+02	2.953125E-02
  | 2.80E-02	-1.481563E+02	1.968750E-02
  | 2.80E-02	-1.464375E+02	2.437500E-02
  | 2.81E-02	-1.498750E+02	3.921875E-02
  | 2.81E-02	-1.470938E+02	2.953125E-02
  | 2.82E-02	-1.436875E+02	1.937500E-02
  | 2.82E-02	-1.464375E+02	1.890625E-02
  | 2.83E-02	-1.453750E+02	1.937500E-02
  | 2.83E-02	-1.416563E+02	2.437500E-02
  | 2.84E-02	-1.406563E+02	1.421875E-02
  | 2.84E-02	-1.406875E+02	1.937500E-02
  | 2.85E-02	-1.376563E+02	1.421875E-02
  | 2.85E-02	-1.336563E+02	9.531250E-03
  | 2.86E-02	-1.336250E+02	1.453125E-02
  | 2.86E-02	-1.335938E+02	-5.781250E-03
  | 2.87E-02	-1.305313E+02	-6.250000E-04
  | 2.87E-02	-1.294063E+02	4.687500E-03
  | 2.88E-02	-1.285313E+02	4.375000E-03
  | 2.88E-02	-1.246563E+02	1.421875E-02
  | 2.89E-02	-1.226563E+02	1.968750E-02
  | 2.89E-02	-1.217188E+02	2.437500E-02
  | 2.90E-02	-1.189063E+02	2.437500E-02
  | 2.90E-02	-1.180000E+02	1.968750E-02
  | 2.91E-02	-1.198438E+02	4.531250E-03
  | 2.91E-02	-1.178125E+02	4.531250E-03
  | 2.92E-02	-1.146875E+02	4.531250E-03
  | 2.92E-02	-1.145313E+02	-5.625000E-03
  | 2.93E-02	-1.125000E+02	-5.625000E-03
  | 2.93E-02	-1.074688E+02	-5.625000E-03
  | 2.94E-02	-1.064063E+02	-5.625000E-03
  | 2.94E-02	-1.054688E+02	-5.625000E-03
  | 2.95E-02	-1.006563E+02	-6.250000E-04
  | 2.95E-02	-9.862500E+01	-1.046875E-02
  | 2.96E-02	-9.562500E+01	-5.468750E-03
  | 2.96E-02	-9.275000E+01	9.531250E-03
  | 2.97E-02	-9.071875E+01	-3.125000E-04
  | 2.97E-02	-8.771875E+01	1.484375E-02
  | 2.98E-02	-8.481250E+01	1.968750E-02
  | 2.98E-02	-8.171875E+01	1.968750E-02
  | 2.99E-02	-7.965625E+01	2.984375E-02
  | 2.99E-02	-7.462500E+01	1.468750E-02
  | 3.00E-02	-6.943750E+01	1.468750E-02
  | 3.00E-02	-6.731250E+01	1.468750E-02
  | 3.01E-02	-6.421875E+01	9.531250E-03
  | 3.01E-02	-6.209375E+01	4.687500E-03
  | 3.02E-02	-6.006250E+01	-3.125000E-04
  | 3.02E-02	-5.615625E+01	9.531250E-03
  | 3.03E-02	-5.521875E+01	9.843750E-03
  | 3.03E-02	-5.418750E+01	9.843750E-03
  | 3.04E-02	-5.131250E+01	4.687500E-03
  | 3.04E-02	-4.837500E+01	9.843750E-03
  | 3.05E-02	-4.531250E+01	1.968750E-02
  | 3.05E-02	-4.446875E+01	4.687500E-03
  | 3.06E-02	-4.143750E+01	4.687500E-03
  | 3.06E-02	-3.637500E+01	4.687500E-03
  | 3.07E-02	-3.250000E+01	-3.125000E-04
  | 3.07E-02	-3.043750E+01	4.531250E-03
  | 3.08E-02	-2.940625E+01	-1.062500E-02
  | 3.08E-02	-2.553125E+01	-1.546875E-02
  | 3.09E-02	-2.253125E+01	-3.125000E-04
  | 3.09E-02	-2.353125E+01	-1.062500E-02
  | 3.10E-02	-2.162500E+01	-2.562500E-02
  | 3.10E-02	-1.790625E+01	-2.609375E-02
  | 3.11E-02	-1.500000E+01	-1.078125E-02
  | 3.11E-02	-1.096875E+01	-1.031250E-02
  | 3.12E-02	-7.343750E+00	-2.125000E-02
  | 3.12E-02	-2.500000E+00	8.750000E-03
  | 3.13E-02	2.500000E+00	1.937500E-02
  | 3.13E-02	6.250000E+00	1.406250E-02
  | 3.14E-02	9.187500E+00	1.328125E-02
  | 3.14E-02	1.118750E+01	2.343750E-02
  | 3.15E-02	1.312500E+01	3.390625E-02
  | 3.15E-02	1.518750E+01	3.281250E-03
  | 3.16E-02	1.921875E+01	1.343750E-02
  | 3.16E-02	2.215625E+01	3.890625E-02
  | 3.17E-02	2.221875E+01	1.906250E-02
  | 3.17E-02	2.715625E+01	1.906250E-02
  | 3.18E-02	3.296875E+01	2.906250E-02
  | 3.18E-02	3.296875E+01	1.906250E-02
  | 3.19E-02	3.390625E+01	1.906250E-02
  | 3.19E-02	3.878125E+01	8.906250E-03
  | 3.20E-02	4.178125E+01	-1.562500E-03
  | 3.20E-02	4.268750E+01	1.375000E-02
  | 3.21E-02	4.659375E+01	3.437500E-03
  | 3.21E-02	4.959375E+01	-7.031250E-03
  | 3.22E-02	5.159375E+01	2.390625E-02
  | 3.22E-02	5.459375E+01	2.453125E-02
  | 3.23E-02	5.762500E+01	1.468750E-02
  | 3.23E-02	6.075000E+01	3.515625E-02
  | 3.24E-02	6.284375E+01	2.484375E-02
  | 3.24E-02	6.584375E+01	4.531250E-03
  | 3.25E-02	6.787500E+01	9.218750E-03
  | 3.25E-02	6.990625E+01	-1.562500E-03
  | 3.26E-02	7.290625E+01	-6.406250E-03
  | 3.26E-02	7.475000E+01	4.531250E-03
  | 3.27E-02	7.671875E+01	4.531250E-03
  | 3.27E-02	7.968750E+01	4.531250E-03
  | 3.28E-02	8.153125E+01	1.000000E-02
  | 3.28E-02	8.246875E+01	2.078125E-02
  | 3.29E-02	8.543750E+01	4.687500E-03
  | 3.29E-02	8.643750E+01	-6.093750E-03
  | 3.30E-02	8.862500E+01	1.531250E-02
  | 3.30E-02	9.284375E+01	1.546875E-02
  | 3.31E-02	9.481250E+01	4.531250E-03
  | 3.31E-02	9.700000E+01	3.031250E-02
  | 3.32E-02	1.001563E+02	8.046875E-02
  | 3.32E-02	1.030313E+02	1.340625E-01
  | 3.33E-02	1.020938E+02	2.181250E-01
  | 3.33E-02	1.030313E+02	3.273438E-01
  | 3.34E-02	1.079375E+02	4.403125E-01
  | 3.34E-02	1.080625E+02	5.385938E-01
  | 3.35E-02	1.060313E+02	6.134375E-01
  | 3.35E-02	1.090000E+02	6.725000E-01
  | 3.36E-02	1.119375E+02	6.914063E-01
  | 3.36E-02	1.129688E+02	6.814063E-01
  | 3.37E-02	1.140313E+02	6.671875E-01
  | 3.37E-02	1.147188E+02	6.129688E-01
  | 3.38E-02	1.168438E+02	5.529688E-01
  | 3.38E-02	1.202188E+02	5.143750E-01
  | 3.39E-02	1.242500E+02	4.407813E-01
  | 3.39E-02	1.244375E+02	3.912500E-01
  | 3.40E-02	1.258438E+02	3.720313E-01
  | 3.40E-02	1.319375E+02	3.523438E-01
  | 3.41E-02	1.330313E+02	3.476563E-01
  | 3.41E-02	1.331875E+02	3.476563E-01
  | 3.42E-02	1.340938E+02	3.675000E-01
  | 3.42E-02	1.340938E+02	3.826563E-01
  | 3.43E-02	1.370938E+02	3.776563E-01
  | 3.43E-02	1.360313E+02	3.728125E-01
  | 3.44E-02	1.370938E+02	3.979688E-01
  | 3.44E-02	1.429688E+02	3.932813E-01
  | 3.45E-02	1.437188E+02	3.684375E-01
  | 3.45E-02	1.438438E+02	3.785938E-01
  | 3.46E-02	1.459688E+02	3.687500E-01
  | 3.46E-02	1.469063E+02	3.482813E-01
  | 3.47E-02	1.468438E+02	3.231250E-01
  | 3.47E-02	1.459375E+02	3.035938E-01
  | 3.48E-02	1.450625E+02	2.826563E-01
  | 3.48E-02	1.468438E+02	2.576563E-01
  | 3.49E-02	1.477500E+02	2.385938E-01
  | 3.49E-02	1.499063E+02	2.032813E-01
  | 3.50E-02	1.517188E+02	2.034375E-01
  | 3.50E-02	1.495625E+02	1.990625E-01
  | 3.51E-02	1.499375E+02	1.689063E-01
  | 3.51E-02	1.518750E+02	1.651563E-01
  | 3.52E-02	1.525313E+02	1.356250E-01
  | 3.52E-02	1.497813E+02	9.968750E-02
  | 3.53E-02	1.490313E+02	6.984375E-02
  | 3.53E-02	1.518438E+02	2.484375E-02
  | 3.54E-02	1.526875E+02	-5.156250E-03
  | 3.54E-02	1.500000E+02	-2.031250E-02
  | 3.55E-02	1.490938E+02	-1.578125E-02
  | 3.55E-02	1.526875E+02	-4.687500E-03
  | 3.56E-02	1.508125E+02	-9.687500E-03
  | 3.56E-02	1.470625E+02	-1.562500E-04
  | 3.57E-02	1.497813E+02	1.515625E-02
  | 3.57E-02	1.487813E+02	4.843750E-03
  | 3.58E-02	1.441250E+02	-4.687500E-04
  | 3.58E-02	1.460625E+02	4.531250E-03
  | 3.59E-02	1.471250E+02	4.531250E-03
  | 3.59E-02	1.461250E+02	4.531250E-03
  | 3.60E-02	1.460938E+02	1.468750E-02
  | 3.60E-02	1.452188E+02	1.468750E-02
  | 3.61E-02	1.460938E+02	-1.562500E-04
  | 3.61E-02	1.439688E+02	1.015625E-02
  | 3.62E-02	1.420313E+02	5.156250E-03
  | 3.62E-02	1.411250E+02	-9.687500E-03
  | 3.63E-02	1.370000E+02	-5.156250E-03
  | 3.63E-02	1.379063E+02	-1.000000E-02
  | 3.64E-02	1.398125E+02	-9.687500E-03
  | 3.64E-02	1.366563E+02	-1.562500E-04
  | 3.65E-02	1.366563E+02	9.375000E-03
  | 3.65E-02	1.394688E+02	9.843750E-03
  | 3.66E-02	1.382500E+02	1.484375E-02
  | 3.66E-02	1.350625E+02	2.437500E-02
  | 3.67E-02	1.328125E+02	2.437500E-02
  | 3.67E-02	1.316875E+02	2.437500E-02
  | 3.68E-02	1.294063E+02	1.937500E-02
  | 3.68E-02	1.271563E+02	9.843750E-03
  | 3.69E-02	1.282188E+02	9.843750E-03
  | 3.69E-02	1.262188E+02	9.375000E-03
  | 3.70E-02	1.251563E+02	-1.562500E-04
  | 3.70E-02	1.252500E+02	-1.562500E-04
  | 3.71E-02	1.213438E+02	4.531250E-03
  | 3.71E-02	1.202813E+02	9.375000E-03
  | 3.72E-02	1.182500E+02	1.968750E-02
  | 3.72E-02	1.163438E+02	5.156250E-03
  | 3.73E-02	1.154063E+02	-4.687500E-03
  | 3.73E-02	1.132500E+02	5.625000E-03
  | 3.74E-02	1.132500E+02	-1.390625E-02
  | 3.74E-02	1.103750E+02	-2.875000E-02
  | 3.75E-02	1.072500E+02	-2.375000E-02
  | 3.75E-02	1.061563E+02	-2.375000E-02
  | 3.76E-02	1.022500E+02	-1.453125E-02
  | 3.76E-02	9.728125E+01	-5.156250E-03
  | 3.77E-02	9.621875E+01	-1.562500E-04
  | 3.77E-02	9.328125E+01	9.062500E-03
  | 3.78E-02	8.943750E+01	4.062500E-03
  | 3.78E-02	8.931250E+01	8.593750E-03
  | 3.79E-02	8.837500E+01	8.593750E-03
  | 3.79E-02	8.743750E+01	-1.046875E-02
  | 3.80E-02	8.212500E+01	3.750000E-03
  | 3.80E-02	8.115625E+01	3.750000E-03
  | 3.81E-02	8.115625E+01	-5.781250E-03
  | 3.81E-02	7.284375E+01	1.328125E-02
  | 3.82E-02	7.187500E+01	1.328125E-02
  | 3.82E-02	7.187500E+01	8.593750E-03
  | 3.83E-02	6.875000E+01	8.593750E-03
  | 3.83E-02	6.587500E+01	1.328125E-02
  | 3.84E-02	6.196875E+01	1.812500E-02
  | 3.84E-02	6.196875E+01	4.062500E-03
  | 3.85E-02	5.809375E+01	-9.375000E-04
  | 3.85E-02	5.218750E+01	8.593750E-03
  | 3.86E-02	5.225000E+01	9.062500E-03
  | 3.86E-02	5.225000E+01	-5.468750E-03
  | 3.87E-02	4.821875E+01	-5.468750E-03
  | 3.87E-02	4.334375E+01	9.062500E-03
  | 3.88E-02	4.228125E+01	-9.375000E-04
  | 3.88E-02	4.021875E+01	-9.375000E-04
  | 3.89E-02	3.431250E+01	1.359375E-02
  | 3.89E-02	3.034375E+01	4.062500E-03
  | 3.90E-02	2.934375E+01	8.593750E-03
  | 3.90E-02	2.743750E+01	1.812500E-02
  | 3.91E-02	2.450000E+01	4.062500E-03
  | 3.91E-02	2.262500E+01	-9.375000E-04
  | 3.92E-02	1.865625E+01	8.593750E-03
  | 3.92E-02	1.375000E+01	4.062500E-03
  | 3.93E-02	1.103125E+01	-5.468750E-03
  | 3.93E-02	8.812500E+00	4.375000E-03
  | 3.94E-02	5.875000E+00	4.531250E-03
  | 3.94E-02	2.375000E+00	-4.687500E-04
  | 3.95E-02	1.875000E-01	4.375000E-03
  | 3.95E-02	1.156250E+00	-4.687500E-04
  | 3.96E-02	-1.562500E+00	4.375000E-03
  | 3.96E-02	-7.531250E+00	4.375000E-03
  | 3.97E-02	-8.437500E+00	-4.687500E-04
  | 3.97E-02	-1.046875E+01	9.375000E-03
  | 3.98E-02	-1.553125E+01	4.218750E-03
  | 3.98E-02	-2.031250E+01	4.218750E-03
  | 3.99E-02	-2.231250E+01	4.218750E-03
  | 3.99E-02	-2.437500E+01	-5.937500E-03
  | 4.00E-02	-3.012500E+01	4.218750E-03
  | 4.00E-02	-3.212500E+01	9.218750E-03
  | 4.01E-02	-3.418750E+01	4.218750E-03
  | 4.01E-02	-3.703125E+01	-5.468750E-03
  | 4.02E-02	-3.903125E+01	-5.781250E-03
  | 4.02E-02	-4.203125E+01	4.218750E-03
  | 4.03E-02	-4.531250E+01	-1.062500E-02
  | 4.03E-02	-5.046875E+01	-1.593750E-02
  | 4.04E-02	-5.331250E+01	4.218750E-03
  | 4.04E-02	-5.465625E+01	4.218750E-03
  | 4.05E-02	-5.981250E+01	-7.812500E-04
  | 4.05E-02	-6.471875E+01	4.218750E-03
  | ];
  | %generar vectores
  | time = datos(:,1);
  | Va = datos(:,2);
  | Ia = datos(:,3);
  | 
  | %variables (Workspace)
  | Ts=time(2)-time(1);
  | Var_corriente = [time Ia];
  | Var_tension = [time Va];
  | tf = time(end);
libraries: spsACCurrentSourceLib x7, spsSeriesRLCBranchLib x4, spsCurrentMeasurementLib x1, spsVoltageMeasurementLib x1, spsACVoltageSourceLib x1, spspowerguiLib x1
settings Model: NumberOfSteps=5  Creator=aj_us  LastModifiedBy=ajust
settings SolverCC: AlgebraicLoopSolver=TrustRegion
settings DataIOCC: LimitDataPoints=on  ReturnWorkspaceOutputs=off
settings OptimizationCC: LifeSpan=inf
settings DebuggingCC: AllowSymbolicDim=off  SFUnexpectedBacktrackingDiag=warning  SFNoUnconditionalDefaultTransitionDiag=warning  SFExecutionAtInitializationDiag=none  SFMachineParentedDataDiag=warning  ArithmeticOperatorsInVariantConditions=warning
settings ModelReferenceCC: PropagateSignalLabelsOutOfModel=off
settings SFSimCC: SimUseLocalCustomCode=off  CustomCodeUndefinedFunction=UseInterfaceOnly
settings RTWCC: RTWUseLocalCustomCode=off
settings CodeAppCC: StateflowObjectComments=on
settings GRTTargetCC: TargetLangStandard=C89/C90 (ANSI)
settings ConfigComp: CovMetricSettings=dw  CovSaveCumulativeToWorkspaceVar=on  CovSaveSingleToWorkspaceVar=on  CovExternalEMLEnable=off
settings SimscapeCC: SimscapeNormalizeSystem=off

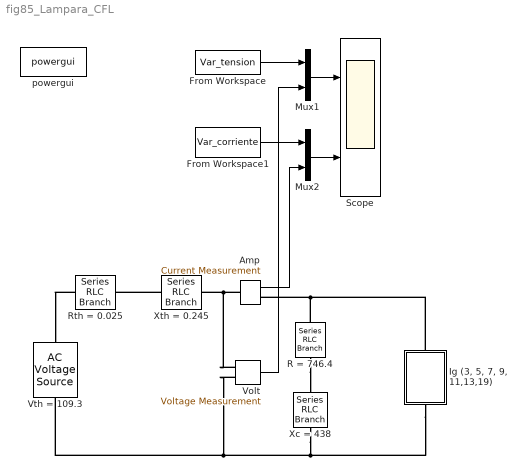
== system fig85_Lampara_CFL ==
  Amp : spsCurrentMeasurementLib/Current Measurement  PhasorSimulation=off  OutputType=Complex  PSBequivalent=0
  From Workspace : FromWorkspace  VariableName=Var_tension  SampleTime=Ts
  From Workspace1 : FromWorkspace  VariableName=Var_corriente  SampleTime=Ts
  "Ig (3, 5, 7, 9, 11,13,19)" : Subsystem
      mask Display: plot(-50,-35,50,50-15,[0,9,18,24,29,30,29,24,18,9,0,-9,-18,-24,-29,-30,-29,-24,-18,-9,0],[30,29,24,18,9,0,-9,-18,-24,-29,-30,-29,-24,-18,-9,0,9,18,24,29,30],[-20 5 5 20 5 5],[2 2 12 2 -8 2],[-50 -30],[0 0],[50,30],[0 0],[45 35 40 40 40],[15 15 15 20 10]);
  Mux1 : Mux  Inputs=2
  Mux2 : Mux  Inputs=2
  R = 746.4 : spsSeriesRLCBranchLib/Series RLC Branch  LConnTagsString=__new0  RConnTagsString=__new0  BranchType=R  Resistance=746.4  Inductance=1e-3  SetiL0=off  InitialCurrent=0  Capacitance=1/(2*pi*60*437.9)  Setx0=off  InitialVoltage=0  Measurements=None
  Rth = 0.025 : spsSeriesRLCBranchLib/Series RLC Branch  LConnTagsString=__new0  RConnTagsString=__new0  BranchType=R  Resistance=0.025  Inductance=1e-3  SetiL0=off  InitialCurrent=0  Capacitance=1/(2*pi*60*437.9)  Setx0=off  InitialVoltage=0  Measurements=None
  Scope : Scope  NumInputPorts=2
  Volt : spsVoltageMeasurementLib/Voltage Measurement  PhasorSimulation=off  OutputType=Complex  PSBequivalent=0
  Vth = 109.3 : spsACVoltageSourceLib/AC Voltage Source  Amplitude=sqrt(2)*109.3  Phase=45.26  Frequency=60  SampleTime=Ts  Measurements=None  BusType=swing  Pref=10e3  Qref=0  Qmin=-inf  Qmax=+inf
  Xc = 438 : spsSeriesRLCBranchLib/Series RLC Branch  LConnTagsString=__new0  RConnTagsString=__new0  BranchType=C  Resistance=758  Inductance=1e-3  SetiL0=off  InitialCurrent=0  Capacitance=1/(2*pi*60*438)  Setx0=off  InitialVoltage=0  Measurements=None
  Xth = 0.245 : spsSeriesRLCBranchLib/Series RLC Branch  LConnTagsString=__new0  RConnTagsString=__new0  BranchType=L  Resistance=758  Inductance=0.245/(2*pi*60)  SetiL0=off  InitialCurrent=0  Capacitance=1/(2*pi*60*437.9)  Setx0=off  InitialVoltage=0  Measurements=None
  powergui : spspowerguiLib/powergui  Priority=1  SimulationMode=Discrete  SampleTime=Ts  frequency=60  Iterations=50  frequencyindice=60  Pbase=100e6  ErrMax=1e-4  UnitsV=kV  UnitsW=MW  buscounter=0  FunctionMessages=off  echomessages=off  EnableUseOfTLC=off  CurrentSourceSwitches=off  DisableSnubberDevices=off  DisableRonSwitches=off  DisableVfSwitches=off  DisplayEquations=off  AutomaticDiscreteSolvers=off  SolverType=Tustin/Backward Euler (TBE)  Interpol=off  ExternalGateDelay=off  methode=off  Ts=10  x0status=blocks  SPID=off  SwTol=0  HookPort=off  NonlinearTolerance=1e-4  nMaxIteration=100  ContinueOnMaxIteration=off  RestoreLinks=warning  ResistiveCurrentMeasurement=off  Frange=[0:2:1000]  Ylog=off  Xlog=off  ShowGrid=on  save=on  variable=ZData  structure=ScopeData  ZoomFFT=off  StartTime=1/60  cycles=1  DisplayStyle=2  fundamental=60  FreqAxis=on  MaxFrequency=1200  frequencyindicesteady=1  RmsSteady=2  display=off
  wires:
  From Workspace1/1 -> Mux2/1
  Mux2/1 -> Scope/2
  Amp/1 -> Mux2/2
  Mux1/1 -> Scope/1
  Volt/1 -> Mux1/2
  From Workspace/1 -> Mux1/1
  connections:
  Amp/LConn1 -- Volt/LConn1 -- Xth = 0.245/RConn1
  Rth = 0.025/LConn1 -- Vth = 109.3/RConn1
  Xth = 0.245/LConn1 -- Rth = 0.025/RConn1
  R = 746.4/RConn1 -- Xc = 438/LConn1
  R = 746.4/LConn1 -- "Ig (3, 5, 7, 9, 11,13,19)"/RConn1 -- Amp/RConn1
  Xc = 438/RConn1 -- Volt/LConn2 -- Vth = 109.3/LConn1 -- "Ig (3, 5, 7, 9, 11,13,19)"/LConn1

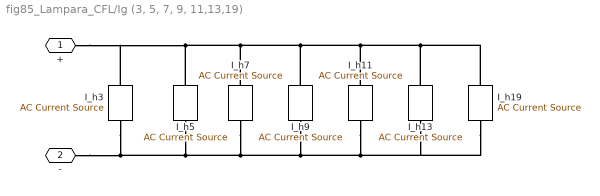
== system fig85_Lampara_CFL/Ig (3, 5, 7, 9, 11,13,19) ==
  I_h11 : spsACCurrentSourceLib/AC Current Source  Amplitude=0.04163  Phase=34.48  Frequency=660  SampleTime=Ts  Measurements=None
      settings: SourceProductBaseCode=PS
  I_h13 : spsACCurrentSourceLib/AC Current Source  Amplitude=0.04255  Phase=19.85  Frequency=13*60  SampleTime=Ts  Measurements=None
      settings: SourceProductBaseCode=PS
  I_h19 : spsACCurrentSourceLib/AC Current Source  Amplitude=0.02406  Phase=0.2031  Frequency=19*60  SampleTime=Ts  Measurements=None
      settings: SourceProductBaseCode=PS
  I_h3 : spsACCurrentSourceLib/AC Current Source  Amplitude=0.151  Phase=44.13  Frequency=180  SampleTime=Ts  Measurements=None
      settings: SourceProductBaseCode=PS
  I_h5 : spsACCurrentSourceLib/AC Current Source  Amplitude=0.1036  Phase=15.42  Frequency=300  SampleTime=Ts  Measurements=None
      settings: SourceProductBaseCode=PS
  I_h7 : spsACCurrentSourceLib/AC Current Source  Amplitude=0.05841  Phase=-1.41  Frequency=420  SampleTime=Ts  Measurements=None
      settings: SourceProductBaseCode=PS
  I_h9 : spsACCurrentSourceLib/AC Current Source  Amplitude=0.03537  Phase=20.15  Frequency=540  SampleTime=Ts  Measurements=None
      settings: SourceProductBaseCode=PS
  + : PMIOPort  Side=Left
  - : PMIOPort  Port=2  Side=Right
  connections:
  I_h13/RConn1 -- I_h19/RConn1 -- I_h11/RConn1 -- I_h9/RConn1 -- I_h7/RConn1 -- I_h3/RConn1 -- +/RConn1 -- I_h5/RConn1
  I_h11/LConn1 -- I_h13/LConn1 -- I_h19/LConn1 -- I_h9/LConn1 -- I_h7/LConn1 -- I_h5/LConn1 -- I_h3/LConn1 -- -/RConn1
